simulink model "HW5Base"  (R2020a)
settings: Solver=VariableStepAuto  StartTime=0.0  StopTime=10.0  RelTol=1e-3
undefined symbols (not defined in the file or in its folder): b, d, d_cg, g, k_m, m, V_1, V_2, V_3, V_4
libraries: shared6dof x1
settings Model: Creator=BAI  LastModifiedBy=BAI

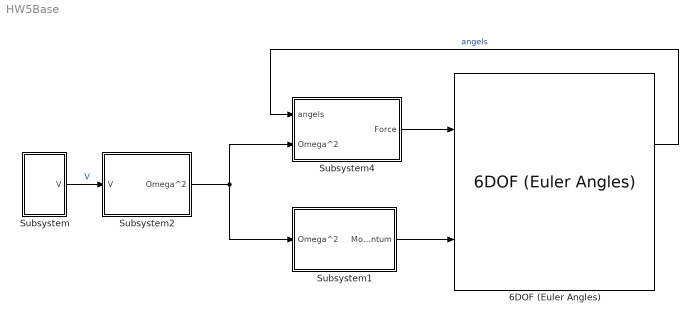
== system HW5Base ==
  6DOF (Euler Angles) : shared6dof/6DOF (Euler Angles)  units=Metric (MKS)  mtype=Fixed  rep=Euler Angles  xme_0=[0 0 0]  Vm_0=[0 0 0]  eul_0=[0 0 0]  pm_0=[0 0 0]  mass_0=1.0  mass_e=0.5  mass_f=2.0  inertia=I  inertia_e=eye(3)  inertia_f=2*eye(3)  k_quat=1.0  vre_flag=on  abi_flag=off  aMode=0  xme_statename=''  Vm_statename=''  eul_statename=''  quat_statename=''  pm_statename=''  mass_statename=''
      settings: SourceProductBaseCode=AE,PW,MT,VE,VP
  Subsystem : Subsystem
  Subsystem1 : Subsystem
  Subsystem2 : Subsystem
  Subsystem4 : Subsystem
  wires:
  Subsystem1/1(Momentum) -> 6DOF (Euler Angles)/2
  Subsystem4/1(Force) -> 6DOF (Euler Angles)/1
  6DOF (Euler Angles)/3 -> Subsystem4/1(angels)  "angels"
  Subsystem2/1(Omega^2) -> Subsystem4/2(Omega^2), Subsystem1/1(Omega^2)
  Subsystem/1(V) -> Subsystem2/1(V)  "V"

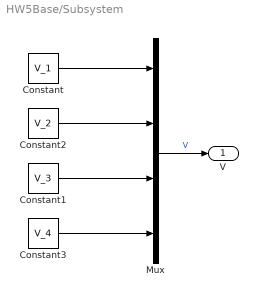
== system HW5Base/Subsystem ==
  Constant : Constant  Value=V_1
  Constant1 : Constant  Value=V_3
  Constant2 : Constant  Value=V_2
  Constant3 : Constant  Value=V_4
  Mux : Mux
  V : Outport
  wires:
  Mux/1 -> V/1  "V"
  Constant/1 -> Mux/1
  Constant3/1 -> Mux/4
  Constant2/1 -> Mux/2
  Constant1/1 -> Mux/3

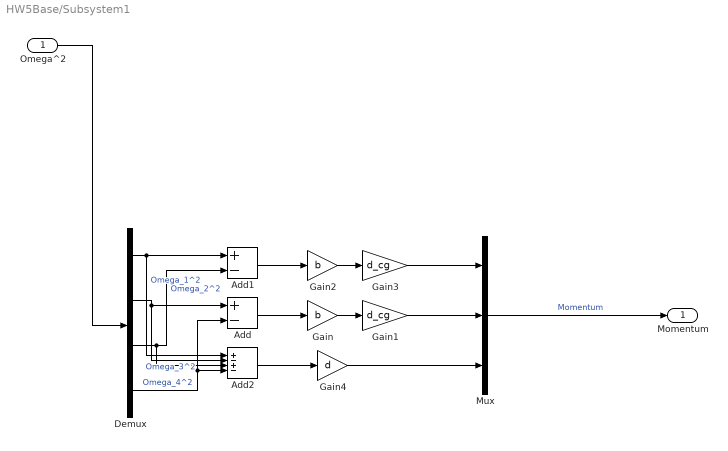
== system HW5Base/Subsystem1 ==
  Omega^2 : Inport
  Add : Sum  Inputs=+-
  Add1 : Sum  Inputs=+-
  Add2 : Sum  Inputs=+-+-
  Demux : Demux
  Gain : Gain  Gain=b
  Gain1 : Gain  Gain=d_cg
  Gain2 : Gain  Gain=b
  Gain3 : Gain  Gain=d_cg
  Gain4 : Gain  Gain=d
  Mux : Mux  Inputs=3
  Momentum : Outport
  wires:
  Gain3/1 -> Mux/1
  Demux/2 -> Add2/2, Add/1  "Omega_3^2"
  Demux/1 -> Add2/1, Add1/1  "Omega_1^2"
  Add2/1 -> Gain4/1
  Demux/3 -> Add2/3, Add1/2  "Omega_2^2"
  Add1/1 -> Gain2/1
  Gain1/1 -> Mux/2
  Demux/4 -> Add2/4, Add/2  "Omega_4^2"
  Gain/1 -> Gain1/1
  Add/1 -> Gain/1
  Gain4/1 -> Mux/3
  Gain2/1 -> Gain3/1
  Omega^2/1 -> Demux/1
  Mux/1 -> Momentum/1  "Momentum"

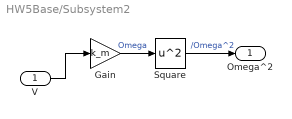
== system HW5Base/Subsystem2 ==
  V : Inport
  Gain : Gain  Gain=k_m
  Square : Math  Operator=square  SaturateOnIntegerOverflow=on
  Omega^2 : Outport
  wires:
  Gain/1 -> Square/1  "Omega"
  V/1 -> Gain/1
  Square/1 -> Omega^2/1  "/Omega^2"

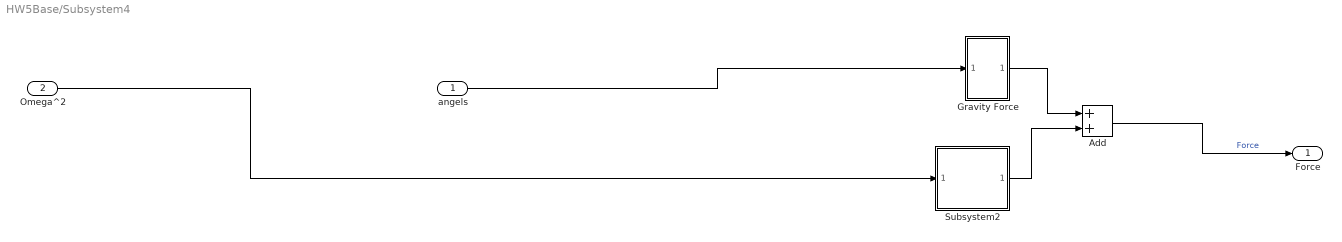
== system HW5Base/Subsystem4 ==
  angels : Inport
  Omega^2 : Inport  Port=2
  Add : Sum
  Gravity Force : Subsystem
  Subsystem2 : Subsystem
  Force : Outport
  wires:
  Gravity Force/1(Out1) -> Add/1
  Subsystem2/1(Thrust1) -> Add/2
  angels/1 -> Gravity Force/1(In1)
  Omega^2/1 -> Subsystem2/1(Omega^2)
  Add/1 -> Force/1  "Force"

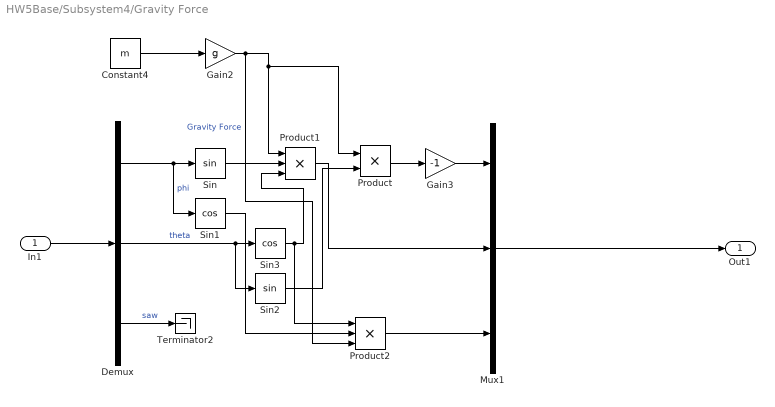
== system HW5Base/Subsystem4/Gravity Force ==
  In1 : Inport
  Constant4 : Constant  Value=m
  Demux : Demux  Outputs=3
  Gain2 : Gain  Gain=g
  Gain3 : Gain  Gain=-1
  Mux1 : Mux  Inputs=3
  Product : Product
  Product1 : Product  Inputs=3
  Product2 : Product  Inputs=3
  Sin : Trigonometry
  Sin1 : Trigonometry  Operator=cos
  Sin2 : Trigonometry
  Sin3 : Trigonometry  Operator=cos
  Terminator2 : Terminator
  Out1 : Outport
  wires:
  Sin3/1 -> Product2/1, Product1/3
  Sin1/1 -> Product2/2
  Gain2/1 -> Product2/3, Product1/1, Product/1  "Gravity Force"
  Demux/3 -> Terminator2/1  "saw"
  Demux/1 -> Sin1/1, Sin/1  "phi"
  Product/1 -> Gain3/1
  Constant4/1 -> Gain2/1
  Demux/2 -> Sin2/1, Sin3/1  "theta"
  Product1/1 -> Mux1/2
  Product2/1 -> Mux1/3
  Sin2/1 -> Product/2
  Sin/1 -> Product1/2
  Gain3/1 -> Mux1/1
  Mux1/1 -> Out1/1
  In1/1 -> Demux/1

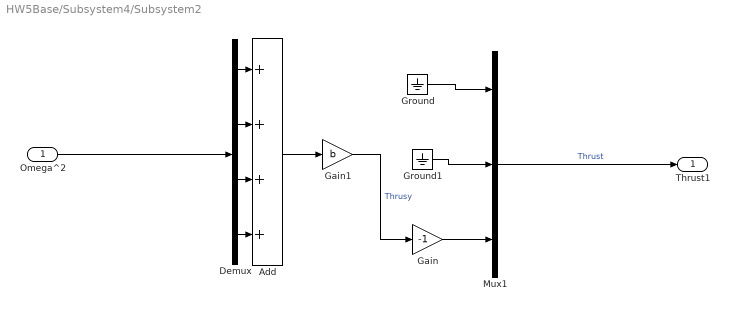
== system HW5Base/Subsystem4/Subsystem2 ==
  Omega^2 : Inport
  Add : Sum  Inputs=++++
  Demux : Demux
  Gain : Gain  Gain=-1
  Gain1 : Gain  Gain=b
  Ground : Ground
  Ground1 : Ground
  Mux1 : Mux  Inputs=3
  Thrust1 : Outport
  wires:
  Ground/1 -> Mux1/1
  Ground1/1 -> Mux1/2
  Mux1/1 -> Thrust1/1  "Thrust"
  Gain1/1 -> Gain/1  "Thrusy"
  Omega^2/1 -> Demux/1
  Demux/1 -> Add/1
  Demux/2 -> Add/2
  Demux/3 -> Add/3
  Demux/4 -> Add/4
  Add/1 -> Gain1/1
  Gain/1 -> Mux1/3
